simulink model "bloques_accion_integral"  (R2021a)
settings: Solver=ode4  StartTime=0.0  StopTime=96  FixedStep=1e-4  RelTol=1e-3
values from neighbouring files (symbols this model uses):
  A = [ ... (first row only)    [disenio_accion_integral.m]
  B = [ B_sb; 0; 0; 0 ]    [disenio_accion_integral.m]
  C = [ ... (first row only)    [disenio_accion_integral.m]
undefined symbols (not defined in the file or in its folder): Hc, Kc, Lc
settings Model: Creator=rocio  LastModifiedBy=rocio

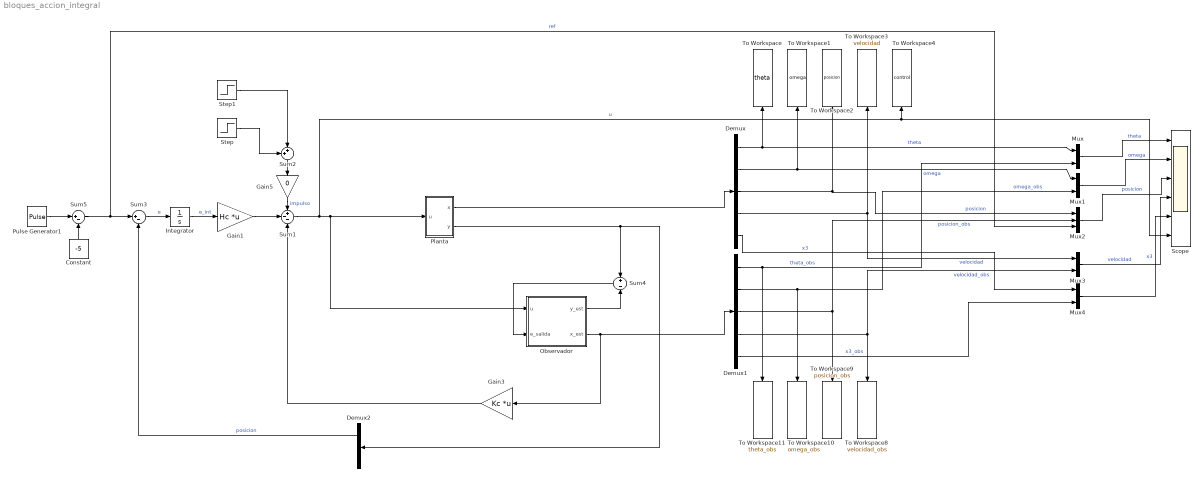
== system bloques_accion_integral ==
  Constant : Constant  Value=-5
  Demux : Demux  Outputs=5
  Demux1 : Demux  Outputs=5
  Demux2 : Demux  Outputs=2
  Gain1 : Gain  Gain=Hc  Multiplication=Matrix(K*u) (u vector)
  Gain3 : Gain  Gain=Kc  Multiplication=Matrix(K*u) (u vector)
  Gain5 : Gain  Gain=0
  Integrator : Integrator
  Mux{,1,3..4} (4 alike) : Mux  Inputs=2
  Mux2 : Mux  Inputs=3
  Observador : Subsystem
  Planta : Subsystem
  Pulse Generator1 : DiscretePulseGenerator  PulseType=Time based  Amplitude=-10  Period=16  PulseWidth=50
  Scope : Scope  NumInputPorts=6
  Step : Step  Time=1.2  After=-1  SampleTime=0
  Step1 : Step  Time=0.8  SampleTime=0
  Sum1 : Sum  Inputs=+--
  Sum2 : Sum  Inputs=++|
  Sum3 : Sum  Inputs=|+-
  Sum4 : Sum  Inputs=+|-
  Sum5 : Sum  Inputs=|+-
  To Workspace : ToWorkspace  VariableName=theta  SampleTime=-1
      settings: Save2DSignal=2-D array (concatenate along first dimension)
  To Workspace1 : ToWorkspace  VariableName=omega  SampleTime=-1
      settings: Save2DSignal=2-D array (concatenate along first dimension)
  To Workspace10 : ToWorkspace  VariableName=omega_obs  SampleTime=-1
      settings: Save2DSignal=2-D array (concatenate along first dimension)
  To Workspace11 : ToWorkspace  VariableName=theta_obs  SampleTime=-1
      settings: Save2DSignal=2-D array (concatenate along first dimension)
  To Workspace2 : ToWorkspace  VariableName=posicion  SampleTime=-1
      settings: Save2DSignal=2-D array (concatenate along first dimension)
  To Workspace3 : ToWorkspace  VariableName=velocidad  SampleTime=-1
      settings: Save2DSignal=2-D array (concatenate along first dimension)
  To Workspace4 : ToWorkspace  VariableName=control  SampleTime=-1
      settings: Save2DSignal=2-D array (concatenate along first dimension)
  To Workspace8 : ToWorkspace  VariableName=velocidad_obs  SampleTime=-1
      settings: Save2DSignal=2-D array (concatenate along first dimension)
  To Workspace9 : ToWorkspace  VariableName=posicion_obs  SampleTime=-1
      settings: Save2DSignal=2-D array (concatenate along first dimension)
  wires:
  Sum1/1 -> To Workspace4/1, Scope/6, Observador/1(u), Planta/1(u)  "u"
  Sum5/1 -> Mux2/3, Sum3/1  "ref"
  Gain3/1 -> Sum1/3
  Step1/1 -> Sum2/2
  Step/1 -> Sum2/1
  Sum2/1 -> Gain5/1
  Gain5/1 -> Sum1/1  "impulso"
  Demux/1 -> Mux/1, To Workspace/1  "theta"
  Demux1/1 -> To Workspace11/1, Mux/2  "theta_obs"
  Demux/2 -> Mux1/1, To Workspace1/1  "omega"
  Demux1/2 -> To Workspace10/1, Mux1/2  "omega_obs"
  Demux/3 -> To Workspace2/1, Mux2/1  "posicion"
  Demux1/3 -> Mux2/2, To Workspace9/1  "posicion_obs"
  Demux/4 -> To Workspace3/1, Mux3/1  "velocidad"
  Demux1/4 -> To Workspace8/1, Mux3/2  "velocidad_obs"
  Mux/1 -> Scope/1  "theta"
  Mux1/1 -> Scope/2  "omega"
  Mux2/1 -> Scope/3  "posicion"
  Mux3/1 -> Scope/4  "velocidad"
  Mux4/1 -> Scope/5  "x3"
  Demux/5 -> Mux4/1  "x3"
  Demux1/5 -> Mux4/2  "x3_obs"
  Observador/2(x_est) -> Gain3/1, Demux1/1
  Sum4/1 -> Observador/2(e_salida)
  Observador/1(y_est) -> Sum4/2
  Planta/1(x) -> Demux/1
  Planta/2(y) -> Sum4/1, Demux2/1
  Gain1/1 -> Sum1/2
  Sum3/1 -> Integrator/1  "e"
  Integrator/1 -> Gain1/1  "e_int"
  Pulse Generator1/1 -> Sum5/1
  Constant/1 -> Sum5/2
  Demux2/1 -> Sum3/2  "posicion"

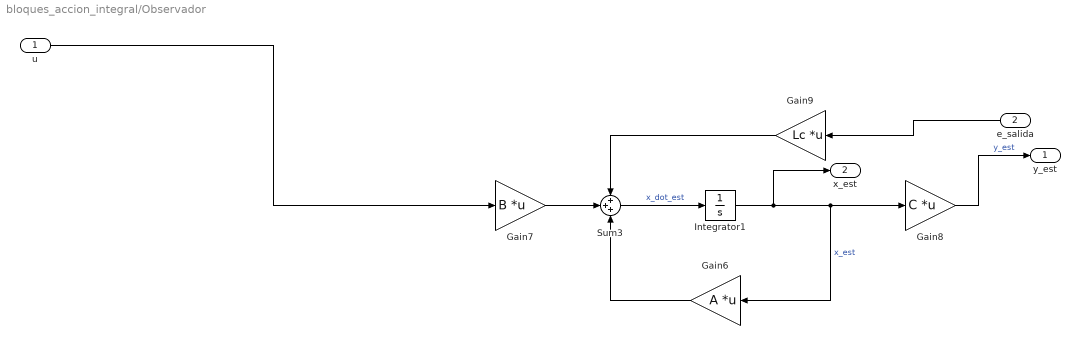
== system bloques_accion_integral/Observador ==
  u : Inport
  e_salida : Inport  Port=2
  Gain6 : Gain  Gain=A  Multiplication=Matrix(K*u) (u vector)
  Gain7 : Gain  Gain=B  Multiplication=Matrix(K*u) (u vector)
  Gain8 : Gain  Gain=C  Multiplication=Matrix(K*u) (u vector)
  Gain9 : Gain  Gain=Lc  Multiplication=Matrix(K*u) (u vector)
  Integrator1 : Integrator
  Sum3 : Sum  Inputs=+++
  y_est : Outport
  x_est : Outport  Port=2
  wires:
  Gain9/1 -> Sum3/1
  u/1 -> Gain7/1
  Sum3/1 -> Integrator1/1  "x_dot_est"
  e_salida/1 -> Gain9/1
  Gain6/1 -> Sum3/3
  Gain8/1 -> y_est/1  "y_est"
  Gain7/1 -> Sum3/2
  Integrator1/1 -> Gain6/1, Gain8/1, x_est/1  "x_est"

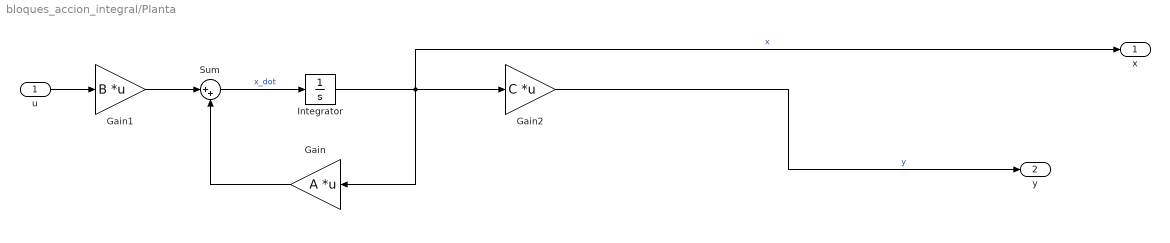
== system bloques_accion_integral/Planta ==
  u : Inport
  Gain : Gain  Gain=A  Multiplication=Matrix(K*u) (u vector)
  Gain1 : Gain  Gain=B  Multiplication=Matrix(K*u) (u vector)
  Gain2 : Gain  Gain=C  Multiplication=Matrix(K*u) (u vector)
  Integrator : Integrator
  Sum : Sum  Inputs=|++
  x : Outport
  y : Outport  Port=2
  wires:
  Gain1/1 -> Sum/1
  u/1 -> Gain1/1
  Gain/1 -> Sum/2
  Integrator/1 -> x/1, Gain2/1, Gain/1  "x"
  Sum/1 -> Integrator/1  "x_dot"
  Gain2/1 -> y/1  "y"
